simulink model "simpleTest"  (R2021a)
settings: Solver=VariableStepAuto  StartTime=0.0  StopTime=10.0  FixedStep=1/20000  RelTol=1e-3
InitFcn:
  | run('init.m');
libraries: mpclib x1
settings Model: Creator=Max  LastModifiedBy=Max

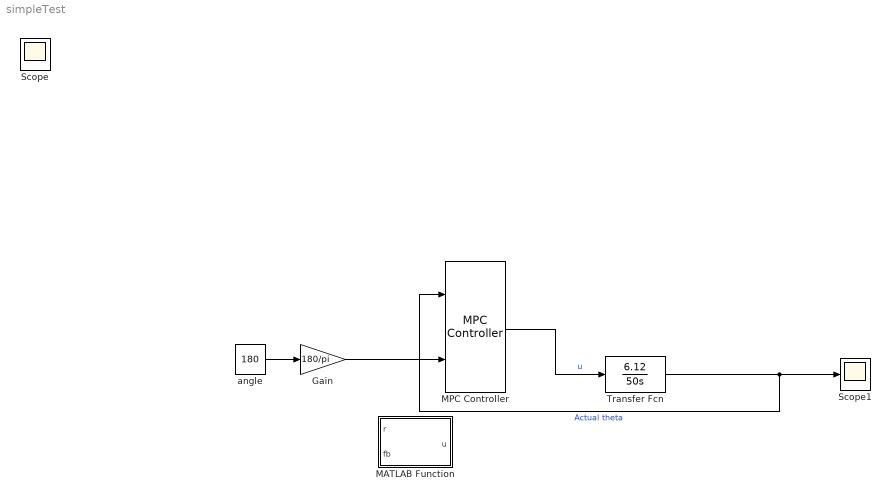
== system simpleTest ==
  Gain : Gain  Gain=180/pi
  MATLAB Function : MATLAB Function  TreatAsAtomicUnit=on
  MPC Controller : mpclib/MPC Controller  SCDEnableBlockLinearizationSpecification=on  is_multiple=0  enable_value=0  return_u0=off  updateMPCinCallerWorkspace=on  md_inport=off  mv_inport=off  uref_inport=off  return_cost=off  return_mvseq=off  return_qpstatus=off  return_xseq=off  return_state=off  return_ovseq=off  state_inport=off  umin_inport=off  umax_inport=off  ymin_inport=off  ymax_inport=off  cc_inport=off  ywt_inport=off  uwt_inport=off  duwt_inport=off  rhoeps_inport=off  pm_inport=off  MaximumP=10  HorizonChoice=FixedHorizon  n_ts=0.001  n_p=10  n_mv=1  n_md=1  n_ud=0  n_mo=1  n_uo=0  BlockDataType=double  SampleTimeInherited=off  switch_inport=off
  Scope1 : Scope
  Transfer Fcn : TransferFcn  Numerator=[6.12]  Denominator=[50 0]
  angle : Constant  Value=180
  Scope : Scope
  wires:
  angle/1 -> Gain/1
  Transfer Fcn/1 -> Scope1/1, MPC Controller/1  "Actual theta"
  MPC Controller/1 -> Transfer Fcn/1  "u"
  Gain/1 -> MPC Controller/2

== matlab function simpleTest/MATLAB Function ==
  data: r input; u output; fb input
function u = MPC(r, fb)

u = 0.01*(r-fb);
